simulink model "validierung"  (R2021a)
settings: Solver=VariableStepAuto  StartTime=0.0  StopTime=time_val  RelTol=1e-3
values from neighbouring files (symbols this model uses):
  Delta = 8e-3    (= 0.008)    [check_output.m]    (also in init.m; init_2.m; temp.m; toolbox_ident.m)
settings Model: Creator=saleh  LastModifiedBy=saleh

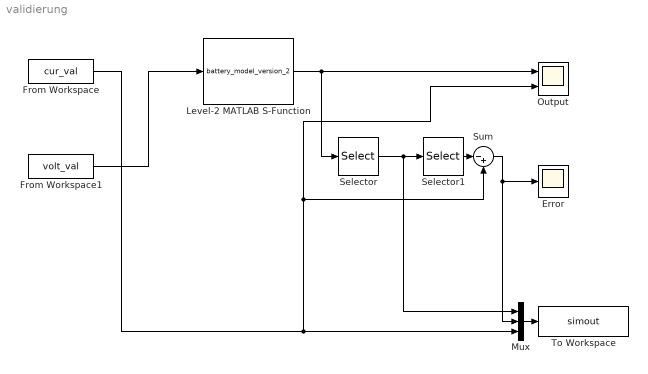
== system validierung ==
  Error : Scope
  From Workspace : FromWorkspace  VariableName=cur_val  SampleTime=Delta
  From Workspace1 : FromWorkspace  VariableName=volt_val  SampleTime=Delta
  Level-2 MATLAB S-Function : M-S-Function  FunctionName=battery_model_version_2  Parameters=x_conv, a, Q_e
  Mux : Mux  Inputs=3
  Output : Scope  NumInputPorts=2
  Selector : Selector  InputPortWidth=4  IndexOptions=Index vector (dialog)  Indices=[1 3]  OutputSizes=1
  Selector1 : Selector  InputPortWidth=2  IndexOptions=Index vector (dialog)  Indices=[1]  OutputSizes=1
  Sum : Sum  Inputs=|-+
  To Workspace : ToWorkspace  VariableName=simout  SampleTime=-1
  wires:
  Level-2 MATLAB S-Function/1 -> Selector/1, Output/1
  Sum/1 -> Mux/2, Error/1
  Selector/1 -> Selector1/1, Mux/1
  Mux/1 -> To Workspace/1
  Selector1/1 -> Sum/1
  From Workspace1/1 -> Level-2 MATLAB S-Function/1
  From Workspace/1 -> Output/2, Sum/2, Mux/3
